simulink model "LQR_simulink_control_client"  (R2024b)
settings: Solver=FixedStepAuto  StartTime=0.0  StopTime=15  FixedStep=0.05  RelTol=1e-3
values from neighbouring files (symbols this model uses):
  Ac = LinSystem.Ac    [LQR_matlab_client_Otacky.m]    (also in LQR_matlab_client_Sily.m; LQR_sync_matlab_client.m; sync_matlab_client.m)
  b_moment = 5.4e-6    (= 5.4e-06)    [LQR_matlab_client_Otacky.m]    (also in LQR_matlab_client_Sily.m; LQR_sync_matlab_client.m; sync_matlab_client.m)
  Bmc = LinSystem.Bmc    [LQR_matlab_client_Otacky.m]    (also in LQR_matlab_client_Sily.m; LQR_sync_matlab_client.m)
  Cc = LinSystem.Cc    [LQR_matlab_client_Otacky.m]    (also in LQR_matlab_client_Sily.m; LQR_sync_matlab_client.m; sync_matlab_client.m)
  Dc = LinSystem.Dc    [LQR_matlab_client_Otacky.m]    (also in LQR_matlab_client_Sily.m; LQR_sync_matlab_client.m; sync_matlab_client.m)
  k_thrust = 2.3e-3    (= 0.0023)    [LQR_matlab_client_Otacky.m]    (also in LQR_matlab_client_Sily.m; LQR_sync_matlab_client.m; sync_matlab_client.m)
  kimot_lqr = Kmot_ex_lqr(:, 17:20)    [LQR_koeficienty.m]
  kpmot_lqr = Kmot_ex_lqr(:, 1:16)    [LQR_koeficienty.m]
  l = 0.2051    [LQR_matlab_client_Otacky.m]    (also in LQR_matlab_client_Sily.m; LQR_sync_matlab_client.m; sync_matlab_client.m)
  Q = 1e-3    (= 0.001)    [LQR_matlab_client_Otacky.m]    (also in LQR_matlab_client_Sily.m; LQR_sync_matlab_client.m; sync_matlab_client.m)
  R = 1e-4    (= 0.0001)    [LQR_matlab_client_Otacky.m]    (also in LQR_matlab_client_Sily.m; LQR_sync_matlab_client.m; sync_matlab_client.m)
  timestep = timeData.TimeStep    [LQR_matlab_client_Otacky.m]    (also in LQR_matlab_client_Sily.m; LQR_sync_matlab_client.m; sync_matlab_client.m)
  Ums_p = [ms2; ms2; ms2; ms2]    [LQR_matlab_client_Otacky.m]    (also in LQR_sync_matlab_client.m)
  Xs_p = [0;0;0; 0;0;0; 0;0; 0;0;0; 0;0;0; 0;0]    [LQR_matlab_client_Otacky.m]    (also in LQR_matlab_client_Sily.m; LQR_sync_matlab_client.m)
undefined symbols (not defined in the file or in its folder): Continuous, Time
libraries: simulink_extras x6, simulink x1, mspfiltlib x1, ctrlSharedLib x1
settings Model: Creator=yaozhong.zhang  LastModifiedBy=Admin
settings DebuggingCC: UnconnectedInputMsg=warning  UnconnectedOutputMsg=warning  UnconnectedLineMsg=warning
settings ModelReferenceCC: EnableRefExpFcnMdlSchedulingChecks=on
settings RTWCC: GPUComputeCapability=3.5

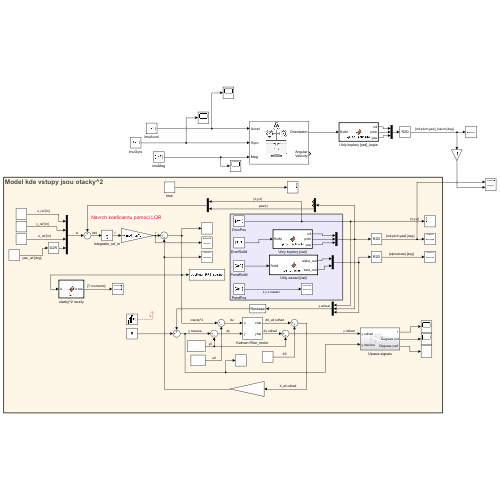
[thumbnail: Simulink's stored preview of the top-level diagram]
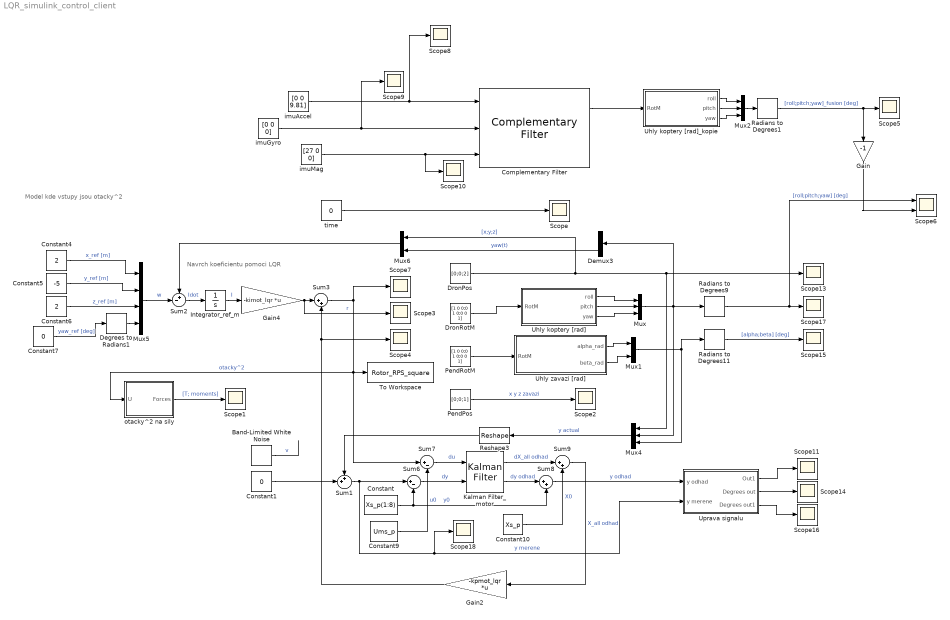
== system LQR_simulink_control_client ==
  note: Model kde vstupy jsou otacky^2
  note: Navrch koeficientu pomoci LQR
  Band-Limited White Noise : simulink/Sources/Band-Limited White Noise  Cov=R*str2num(timestep)  Ts=str2num(timestep)  seed=[23341]
  Complementary Filter : mspfiltlib/Complementary Filter  DispRefFrame=NED  OrientationFormat=Rotation matrix  AccelerometerGain=0.01  HasMagnetometer=on  MagnetometerGain=0.05  SimulateUsing=Interpreted execution
  Constant : Constant  Value=Xs_p(1:8)
  Constant1 : Constant  Value=0
  Constant10 : Constant  Value=Xs_p
  Constant4 : Constant  Value=2
  Constant5 : Constant  Value=-5
  Constant6 : Constant  Value=2
  Constant7 : Constant  Value=0
  Constant9 : Constant  Value=Ums_p
  Degrees to Radians1 : simulink_extras/Transformations/Degrees to Radians
  Demux3 : Demux  Outputs=3
  DronPos : Constant  Value=[0;0;2]  SampleTime=-1
  DronRotM : Constant  Value=[1 0 0;0 1 0;0 0 1]  SampleTime=-1
  Gain : Gain  Gain=-1
  Gain2 : Gain  Gain=-kpmot_lqr  Multiplication=Matrix(K*u)
  Gain4 : Gain  Gain=-kimot_lqr  Multiplication=Matrix(K*u)
  Integrator_ref_m : Integrator  InitialCondition=[1.54346369058432e-13;3.91010801614727e-12;-37.6161056972213;-9.51802609193794e-14]
  Kalman Filter_motor : ctrlSharedLib/Kalman Filter  TimeDomain=Continuous-Time  UseCurrentEstimator=on  ModelSource=Individual A, B, C, D matrices  ModelSourceVariable=ss(0.95,1,1,0,1)  A=Ac  B=Bmc  C=Cc  D=Dc  NumberOfStates=1  NumberOfInputs=1  NumberOfOutputs=1  InitialEstimateSource=Dialog  X0=[0;0;2; 0;0;0; 0;0; 0;0;0; 0;0;0; 0;0]  P0=10  UseK=off  UseGH=off  NumberOfProcessNoiseInputs=1  G=1  TimeInvariantG=on  H=0  TimeInvariantH=on  Q=diag(Q*ones(16,1))  TimeInvariantQ=on  R=diag(R*ones(8,1))  TimeInvariantR=on  N=0  TimeInvariantN=on  AddInputPort=on  AddEnablePort=off  OutputEstimatedY=on  OutputP=off  Ts=-1
  Mux : Mux  Inputs=3
  Mux1 : Mux  Inputs=2
  Mux2 : Mux  Inputs=3
  Mux4 : Mux  Inputs=3
  Mux5 : Mux
  Mux6 : Mux  Inputs=2
  PendPos : Constant  Value=[0;0;1]  SampleTime=-1
  PendRotM : Constant  Value=[1 0 0;0 1 0;0 0 1]  SampleTime=-1
  Radians to Degrees1 : simulink_extras/Transformations/Radians to Degrees
  Radians to Degrees11 : simulink_extras/Transformations/Radians to Degrees
  Radians to Degrees9 : simulink_extras/Transformations/Radians to Degrees
  Reshape3 : Reshape  OutputDimensionality=Customize  OutputDimensions=[8,1]
  Scope{,1..5,7..11,13..18} (17 alike) : Scope
  Scope6 : Scope  NumInputPorts=2
  Sum1 : Sum  Inputs=++|
  Sum2 : Sum  Inputs=+-|
  Sum3 : Sum  Inputs=|++
  Sum6 : Sum  Inputs=|+-
  Sum7 : Sum  Inputs=|+-
  Sum8 : Sum  Inputs=|++
  Sum9 : Sum  Inputs=|++
  To Workspace : ToWorkspace  VariableName=Rotor_RPS_square  SampleTime=-1
  Uhly koptery [rad] : MATLAB Function  TreatAsAtomicUnit=on
  Uhly koptery [rad]_kopie : MATLAB Function  TreatAsAtomicUnit=on
  Uhly zavazi [rad] : MATLAB Function  TreatAsAtomicUnit=on
  Uprava signalu : Subsystem
  imuAccel : Constant  Value=[0 0 9.81]  VectorParams1D=off  SampleTime=-1
  imuGyro : Constant  Value=[0 0 0]  VectorParams1D=off  SampleTime=-1
  imuMag : Constant  Value=[27 0 0]  VectorParams1D=off  SampleTime=-1
  otacky^2 na sily : MATLAB Function  TreatAsAtomicUnit=on
  time : Constant  Value=0  SampleTime=-1
  wires:
  Uhly koptery [rad]/2(pitch) -> Mux/2
  Uhly koptery [rad]/1(roll) -> Mux/1
  Uhly koptery [rad]/3(yaw) -> Mux/3
  PendPos/1 -> Scope2/1  "x y z zavazi"
  DronRotM/1 -> Uhly koptery [rad]/1(RotM)
  PendRotM/1 -> Uhly zavazi [rad]/1(RotM)
  Uhly zavazi [rad]/1(alpha_rad) -> Mux1/1
  Uhly zavazi [rad]/2(beta_rad) -> Mux1/2
  time/1 -> Scope/1
  Mux6/1 -> Sum2/1
  Gain2/1 -> Scope4/1, Sum3/2
  Sum2/1 -> Integrator_ref_m/1  "Idot"
  Constant5/1 -> Mux5/2  "y_ref [m]"
  Constant6/1 -> Mux5/3  "z_ref [m]"
  Uprava signalu/1(Out1) -> Scope11/1
  Radians to Degrees11/1 -> Scope15/1  "[alpha;beta] [deg]"
  Mux/1 -> Demux3/1, Radians to Degrees9/1, Mux4/2
  Mux4/1 -> Reshape3/1  "y actual"
  Uprava signalu/3(Degrees out1) -> Scope16/1
  Constant4/1 -> Mux5/1  "x_ref [m]"
  Integrator_ref_m/1 -> Gain4/1  "I"
  Demux3/3 -> Mux6/2  "yaw(t)"
  Uprava signalu/2(Degrees out) -> Scope14/1
  Degrees to Radians1/1 -> Mux5/4
  Constant7/1 -> Degrees to Radians1/1  "yaw_ref [deg]"
  DronPos/1 -> Scope13/1, Mux4/1, Mux6/1  "[x;y;z]"
  Mux5/1 -> Sum2/2  "w"
  Mux1/1 -> Mux4/3, Radians to Degrees11/1
  Radians to Degrees9/1 -> Scope6/1, Scope17/1  "[roll;pitch;yaw] [deg]"
  otacky^2 na sily/1(Forces) -> Scope1/1  "[T; moments]"
  Constant/1 -> Sum8/2, Sum6/2  "y0"
  Sum6/1 -> Kalman Filter_motor/2  "dy"
  Sum9/1 -> Gain2/1  "X_all odhad"
  Band-Limited White Noise/1 -> ?  "v"
  Reshape3/1 -> Sum1/1
  Kalman Filter_motor/1 -> Sum9/1  "dX_all odhad"
  Sum7/1 -> Kalman Filter_motor/1  "du"
  Sum8/1 -> Uprava signalu/1(y odhad)  "y odhad"
  Constant10/1 -> Sum9/2  "X0"
  Kalman Filter_motor/2 -> Sum8/1  "dy odhad"
  Constant9/1 -> Sum7/2  "u0"
  Sum1/1 -> Sum6/1, Uprava signalu/2(y merene), Scope18/1  "y merene"
  Gain4/1 -> Scope3/1, Sum3/1  "r"
  Sum3/1 -> Sum7/1, otacky^2 na sily/1(U), To Workspace/1, Scope7/1  "otacky^2"
  Constant1/1 -> Sum1/2
  imuAccel/1 -> Scope8/1, Complementary Filter/1
  imuGyro/1 -> Scope9/1, Complementary Filter/2
  Complementary Filter/1 -> Uhly koptery [rad]_kopie/1(RotM)
  Radians to Degrees1/1 -> Gain/1, Scope5/1  "[roll;pitch;yaw]_fusion [deg]"
  Mux2/1 -> Radians to Degrees1/1
  Uhly koptery [rad]_kopie/2(pitch) -> Mux2/2
  Uhly koptery [rad]_kopie/3(yaw) -> Mux2/3
  Uhly koptery [rad]_kopie/1(roll) -> Mux2/1
  Gain/1 -> Scope6/2
  imuMag/1 -> Scope10/1, Complementary Filter/3

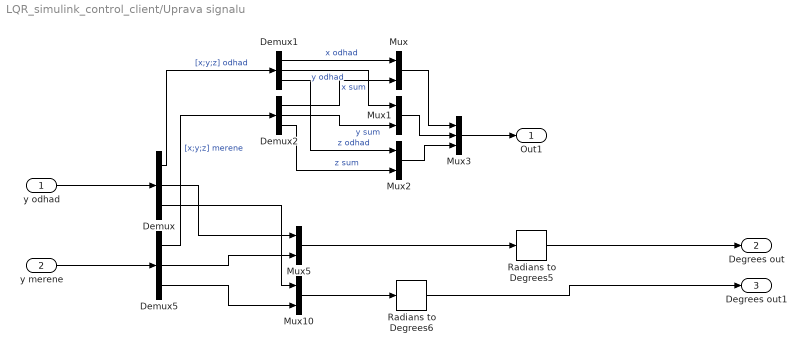
== system LQR_simulink_control_client/Uprava signalu ==
  y odhad : Inport
  y merene : Inport  Port=2
  Demux{,1..2,5} (4 alike) : Demux  Outputs=3
  Mux{,1..2,5,10} (5 alike) : Mux  Inputs=2
  Mux3 : Mux  Inputs=3
  Radians to Degrees5 : simulink_extras/Transformations/Radians to Degrees
  Radians to Degrees6 : simulink_extras/Transformations/Radians to Degrees
  Out1 : Outport
  Degrees out : Outport  Port=2
  Degrees out1 : Outport  Port=3
  wires:
  Demux5/3 -> Mux10/2
  Demux/3 -> Mux10/1
  Mux5/1 -> Radians to Degrees5/1
  Demux/2 -> Mux5/1
  Demux5/2 -> Mux5/2
  Demux5/1 -> Demux2/1  "[x;y;z] merene"
  Demux/1 -> Demux1/1  "[x;y;z] odhad"
  Mux10/1 -> Radians to Degrees6/1
  y odhad/1 -> Demux/1
  Radians to Degrees6/1 -> Degrees out1/1
  Radians to Degrees5/1 -> Degrees out/1
  y merene/1 -> Demux5/1
  Demux1/1 -> Mux/1  "x odhad"
  Demux2/1 -> Mux/2  "x sum"
  Demux1/2 -> Mux1/1  "y odhad"
  Demux2/2 -> Mux1/2  "y sum"
  Mux/1 -> Mux3/1
  Mux1/1 -> Mux3/2
  Mux2/1 -> Mux3/3
  Demux1/3 -> Mux2/1  "z odhad"
  Demux2/3 -> Mux2/2  "z sum"
  Mux3/1 -> Out1/1

== matlab function LQR_simulink_control_client/Uhly zavazi [rad] ==
  data: RotM input; alpha_rad output; beta_rad output
function [alpha_rad, beta_rad] = pend_orient(RotM)
% Расчет углов альфа и бета маятника

% Вектор маятника
rope_vector = RotM * [0; 0; -1];

% Расчет угла альфа
rope_vector_xz = rope_vector([1, 3]); % Компоненты x и z
z_axis = [0; -1];
cos_alpha = dot(rope_vector_xz, z_axis) / (norm(rope_vector_xz) * norm(z_axis));
cos_alpha = max(-1, min(1, cos_alpha)); % Ограничиваем в диапазоне [-1, 1]
alpha = acos(cos_alpha);
if rope_vector(1) < 0
    alpha = -alpha;
end

% Расчет угла бета
rope_vector_xz_3 = [rope_vector(1); 0; rope_vector(3)];
cos_beta = dot(rope_vector, rope_vector_xz_3) / (norm(rope_vector) * norm(rope_vector_xz_3));
cos_beta = max(-1, min(1, cos_beta)); % Ограничиваем в диапазоне [-1, 1]
beta = acos(cos_beta);
if rope_vector(2) < 0
    beta = -beta;
end

% Округляем до 5 знаков после запятой
% alpha_rad = round(alpha, 5); %[rad]
% beta_rad = round(beta, 5); %[rad]
alpha_rad = alpha;
beta_rad = beta;

== matlab function LQR_simulink_control_client/Uhly koptery [rad]_kopie ==
  data: RotM input; roll output; pitch output; yaw output
function [roll, pitch, yaw] = quad_attitude(RotM)
% matice rotace koptery z Python, vuci svetu!!!
% rotm2eul prevadi na Eulerove uhly
radians = rotm2eul(RotM, 'ZYX'); % pouzivam poradi ZYX

% roll = kolem x, pitch = kolem y, yaw = kolem z
yaw = radians(1);
pitch = radians(2);
roll = radians(3);
end

== matlab function LQR_simulink_control_client/Uhly koptery [rad] ==
  data: RotM input; roll output; pitch output; yaw output
function [roll, pitch, yaw] = quad_attitude(RotM)
% matice rotace koptery z Python, vuci svetu!!!
% rotm2eul prevadi na Eulerove uhly
radians = rotm2eul(RotM, 'ZYX'); % pouzivam poradi ZYX

% roll = kolem x, pitch = kolem y, yaw = kolem z
yaw = radians(1);
pitch = radians(2);
roll = radians(3);
end

== matlab function LQR_simulink_control_client/otacky^2 na sily ==
  data: U input; Forces output; l parameter; b_moment parameter; k_thrust parameter
function Forces = fcn(U, l, b_moment, k_thrust)
U1 = U(1);
U2 = U(2);
U3 = U(3);
U4 = U(4);

T = k_thrust*(U1 + U2 + U3 + U4);
Tau_phi = k_thrust*l*(U1 - U2 - U3 + U4);
Tau_theta = -k_thrust*l*(U1 + U2 - U3 - U4);
Tau_psi = b_moment*(U1 - U2 + U3 - U4);

Forces = [T; Tau_phi; Tau_theta; Tau_psi];
